simulink model "clark_nibianhuan"  (R2024b)
settings: Solver=VariableStepAuto  StartTime=0.0  StopTime=10.0  RelTol=1e-3
settings Model: Creator=罗芳成  LastModifiedBy=罗芳成

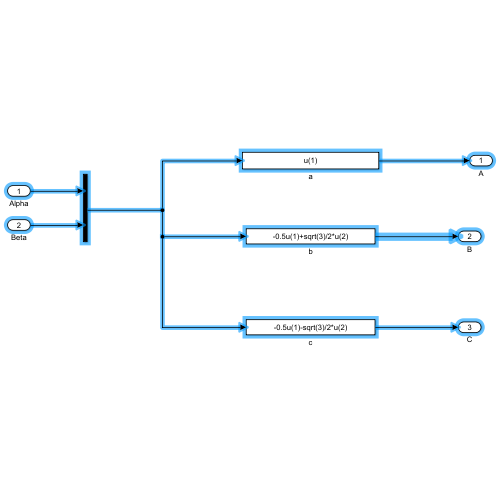
[thumbnail: Simulink's stored preview of the top-level diagram]
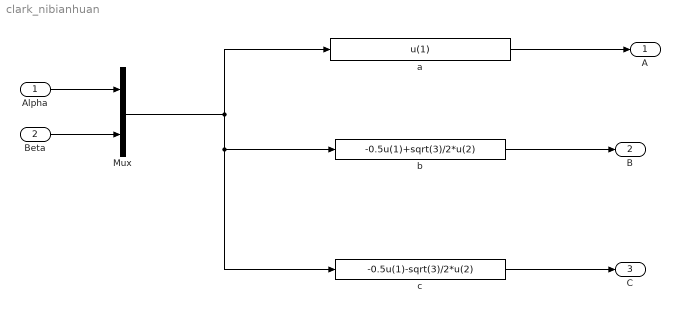
== system clark_nibianhuan ==
  Alpha : Inport
  Beta : Inport  Port=2
  Mux : Mux  Inputs=2
  a : Fcn  Expr=u(1)
  b : Fcn  Expr=-0.5u(1)+sqrt(3)/2*u(2)
  c : Fcn  Expr=-0.5u(1)-sqrt(3)/2*u(2)
  A : Outport
  B : Outport  Port=2
  C : Outport  Port=3
  wires:
  c/1 -> C/1
  a/1 -> A/1
  Mux/1 -> a/1, c/1, b/1
  Alpha/1 -> Mux/1
  Beta/1 -> Mux/2
  b/1 -> B/1
